simulink model "CubaModel"  (R2016a)
settings: Solver=FixedStepAuto  StartTime=0.0  StopTime=3  FixedStep=0.001  RelTol=1e-3
values from neighbouring files (symbols this model uses):
  C_K = 1.02e-3    (= 0.00102)    [initSimulink.m]
  C_R = 0.05e-3    (= 5e-05)    [initSimulink.m]
  g = 9.81    [calculateH.m]    (also in initSimulink.m)
  K_D = 1.8206    [initSimulink.m]
  K_I = 1.4006    [initSimulink.m]
  K_P = 6.4842    [initSimulink.m]
  l_AB = 0.075    [initSimulink.m]
  l_AS = 0.085    [initSimulink.m]
  m_K = 0.419    [initSimulink.m]
  m_R = 0.204    [initSimulink.m]
  O_G_A = O_b_A + m_w * l^2    (= 0.0048139)    [calculateH.m]    (also in initSimulink.m = 0.0044875)
  O_R_B = 0.57e-3    (= 0.00057)    [initSimulink.m]
  phi_K0 = degtorad(0)    [initSimulink.m]
  phi_K__d0 = degtorad(0)    [initSimulink.m]
  phi_R0 = degtorad(0)    [initSimulink.m]
  phi_R__d0 = degtorad(0)    [initSimulink.m]
  T_M_e = 5.5e-4    (= 0.00055)    [initSimulink.m]
  T_M_m = 12.4e-3    (= 0.0124)    [initSimulink.m]
settings Model: Creator=michael  LastModifiedBy=ich

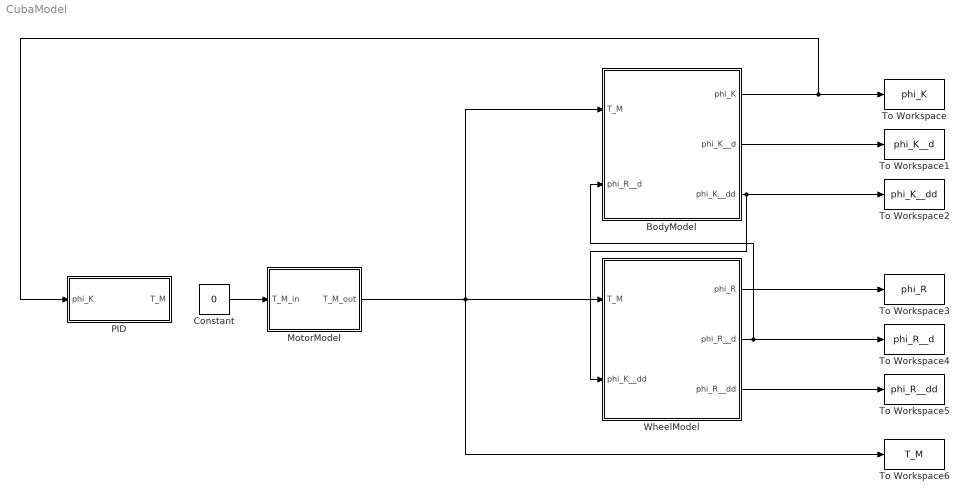
== system CubaModel ==
  BodyModel : Subsystem
  Constant : Constant  Value=0
  "MotorModel " : Subsystem
  PID : Subsystem
  To Workspace : ToWorkspace  VariableName=phi_K  SampleTime=-1
  To Workspace1 : ToWorkspace  VariableName=phi_K__d  SampleTime=-1
  To Workspace2 : ToWorkspace  VariableName=phi_K__dd  SampleTime=-1
  To Workspace3 : ToWorkspace  VariableName=phi_R  SampleTime=-1
  To Workspace4 : ToWorkspace  VariableName=phi_R__d  SampleTime=-1
  To Workspace5 : ToWorkspace  VariableName=phi_R__dd  SampleTime=-1
  To Workspace6 : ToWorkspace  VariableName=T_M  SampleTime=-1
  WheelModel : Subsystem
  wires:
  WheelModel/2(phi_R__d) -> To Workspace4/1, BodyModel/2(phi_R__d)
  BodyModel/3(phi_K__dd) -> To Workspace2/1, WheelModel/2(phi_K__dd)
  BodyModel/1(phi_K) -> PID/1(phi_K), To Workspace/1
  BodyModel/2(phi_K__d) -> To Workspace1/1
  WheelModel/1(phi_R) -> To Workspace3/1
  WheelModel/3(phi_R__dd) -> To Workspace5/1
  "MotorModel "/1(T_M_out) -> BodyModel/1(T_M), WheelModel/1(T_M), To Workspace6/1
  Constant/1 -> "MotorModel "/1(T_M_in)

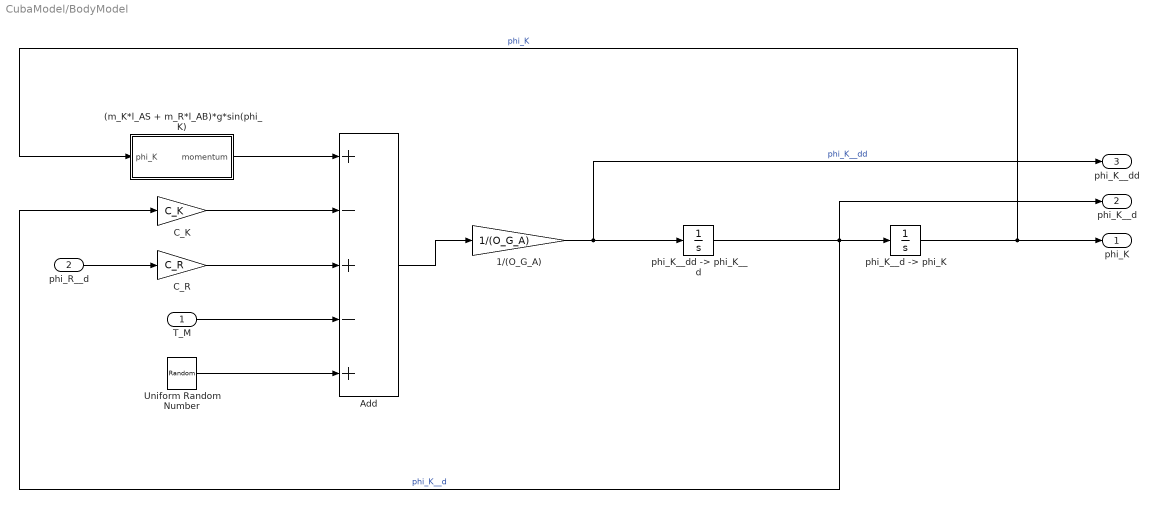
== system CubaModel/BodyModel ==
  T_M : Inport
  phi_R__d : Inport  Port=2
  (m_K*l_AS + m_R*l_AB)*g*sin(phi_K) : Subsystem
  1/(O_G_A) : Gain  Gain=1/(O_G_A)
  Add : Sum  Inputs=+-+-+
  C_K : Gain  Gain=C_K
  C_R : Gain  Gain=C_R
  Uniform Random Number : UniformRandomNumber  Minimum=-0.01  Maximum=0.01  SampleTime=0.001
  "phi_K__d -> phi_K" : Integrator  InitialCondition=phi_K0
  "phi_K__dd -> phi_K__d" : Integrator  InitialCondition=phi_K__d0
  phi_K : Outport
  phi_K__d : Outport  Port=2
  phi_K__dd : Outport  Port=3
  wires:
  T_M/1 -> Add/4
  C_R/1 -> Add/3
  C_K/1 -> Add/2
  (m_K*l_AS + m_R*l_AB)*g*sin(phi_K)/1(momentum) -> Add/1
  phi_R__d/1 -> C_R/1
  Add/1 -> 1/(O_G_A)/1
  1/(O_G_A)/1 -> phi_K__dd/1, "phi_K__dd -> phi_K__d"/1  "phi_K__dd"
  "phi_K__dd -> phi_K__d"/1 -> C_K/1, phi_K__d/1, "phi_K__d -> phi_K"/1  "phi_K__d"
  "phi_K__d -> phi_K"/1 -> phi_K/1, (m_K*l_AS + m_R*l_AB)*g*sin(phi_K)/1(phi_K)  "phi_K"
  Uniform Random Number/1 -> Add/5

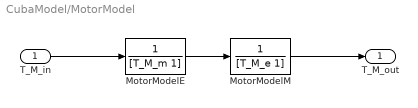
== system CubaModel/MotorModel  ==
  T_M_in : Inport
  MotorModelE : TransferFcn  Denominator=[T_M_m 1]
  MotorModelM : TransferFcn  Denominator=[T_M_e 1]
  T_M_out : Outport
  wires:
  MotorModelE/1 -> MotorModelM/1
  T_M_in/1 -> MotorModelE/1
  MotorModelM/1 -> T_M_out/1

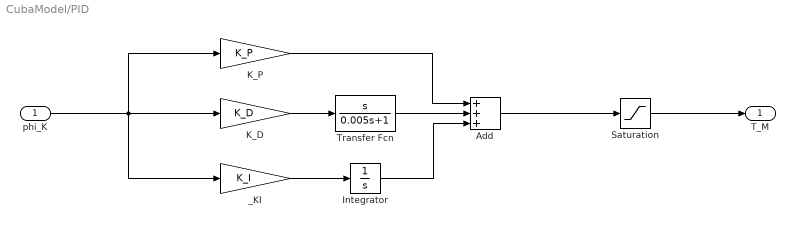
== system CubaModel/PID ==
  phi_K : Inport
  Add : Sum  Inputs=+++
  Integrator : Integrator
  K_D : Gain  Gain=K_D
  K_P : Gain  Gain=K_P
  Saturation : Saturate  UpperLimit=0.1  LowerLimit=-0.1
  Transfer Fcn : TransferFcn  Numerator=[1 0]  Denominator=[0.005 1]
  _KI : Gain  Gain=K_I
  T_M : Outport
  wires:
  phi_K/1 -> _KI/1, K_P/1, K_D/1
  _KI/1 -> Integrator/1
  Add/1 -> Saturation/1
  K_D/1 -> Transfer Fcn/1
  Integrator/1 -> Add/3
  K_P/1 -> Add/1
  Transfer Fcn/1 -> Add/2
  Saturation/1 -> T_M/1

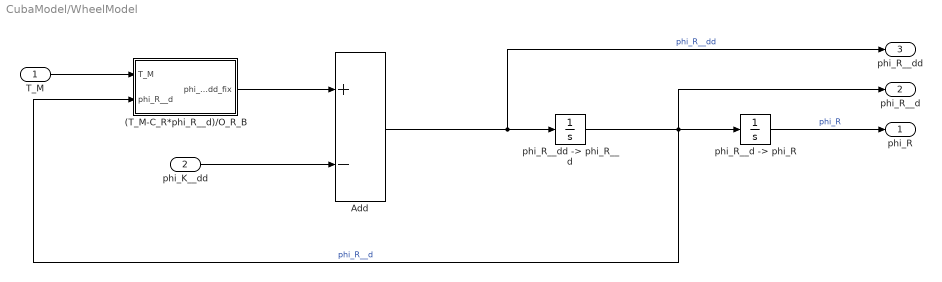
== system CubaModel/WheelModel ==
  T_M : Inport
  phi_K__dd : Inport  Port=2
  (T_M-C_R*phi_R__d)/O_R_B : Subsystem
  Add : Sum  Inputs=+-
  "phi_R__d -> phi_R" : Integrator  InitialCondition=phi_R0
  "phi_R__dd -> phi_R__d" : Integrator  InitialCondition=phi_R__d0
  phi_R : Outport
  phi_R__d : Outport  Port=2
  phi_R__dd : Outport  Port=3
  wires:
  phi_K__dd/1 -> Add/2
  Add/1 -> phi_R__dd/1, "phi_R__dd -> phi_R__d"/1  "phi_R__dd"
  "phi_R__dd -> phi_R__d"/1 -> phi_R__d/1, (T_M-C_R*phi_R__d)/O_R_B/2(phi_R__d), "phi_R__d -> phi_R"/1  "phi_R__d"
  (T_M-C_R*phi_R__d)/O_R_B/1(phi_R__dd_fix) -> Add/1
  T_M/1 -> (T_M-C_R*phi_R__d)/O_R_B/1(T_M)
  "phi_R__d -> phi_R"/1 -> phi_R/1  "phi_R"

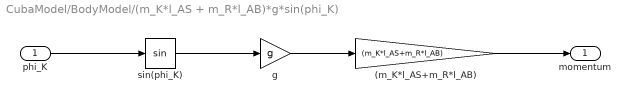
== system CubaModel/BodyModel/(m_K*l_AS + m_R*l_AB)*g*sin(phi_K) ==
  phi_K : Inport
  (m_K*l_AS+m_R*l_AB) : Gain  Gain=(m_K*l_AS+m_R*l_AB)
  g : Gain  Gain=g
  sin(phi_K) : Trigonometry
  momentum : Outport
  wires:
  sin(phi_K)/1 -> g/1
  phi_K/1 -> sin(phi_K)/1
  g/1 -> (m_K*l_AS+m_R*l_AB)/1
  (m_K*l_AS+m_R*l_AB)/1 -> momentum/1

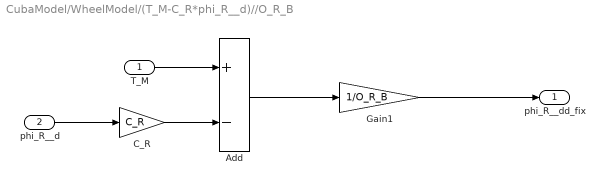
== system CubaModel/WheelModel/(T_M-C_R*phi_R__d)//O_R_B ==
  T_M : Inport
  phi_R__d : Inport  Port=2
  Add : Sum  Inputs=+-
  C_R : Gain  Gain=C_R
  Gain1 : Gain  Gain=1/O_R_B
  phi_R__dd_fix : Outport
  wires:
  T_M/1 -> Add/1
  phi_R__d/1 -> C_R/1
  C_R/1 -> Add/2
  Add/1 -> Gain1/1
  Gain1/1 -> phi_R__dd_fix/1
